simulink model "autosar_swc_expfcns"  (R2022b)
settings: Solver=FixedStepDiscrete  StartTime=0.0  StopTime=0.025  FixedStep=1  MaxStep=.0001  RelTol=1e-3  EnableMultiTasking=on
undefined symbols (not defined in the file): DiscIntNeverNeededParam
settings Model: Creator=The MathWorks, Inc.  LastModifiedBy=The MathWorks, Inc.
settings SolverCC: AlgebraicLoopSolver=TrustRegion  MaxZcPerStep=1
settings DataIOCC: LimitDataPoints=on  SaveFormat=Array  SaveOutput=off  SaveTime=off  ReturnWorkspaceOutputs=off
settings OptimizationCC: DefaultParameterBehavior=Inlined  InlineInvariantSignals=on  EnhancedBackFolding=on  ExpressionDepthLimit=2147483647  StateBitsets=on  DataBitsets=on  ZeroExternalMemoryAtStartup=off  ZeroInternalMemoryAtStartup=off  NoFixptDivByZeroProtection=on  EfficientFloat2IntCast=on  EfficientMapNaN2IntZero=off  LifeSpan=1  BufferReusableBoundary=off  EfficientTunableParamExpr=on
settings DebuggingCC: SigSpecEnsureSampleTimeMsg=none  UnconnectedInputMsg=warning  UnconnectedOutputMsg=warning  UnconnectedLineMsg=warning  BusObjectLabelMismatch=none  AllowSymbolicDim=off  StateNameClashWarn=warning  PregeneratedLibrarySubsystemCodeDiagnostic=none  StrictBusMsg=ErrorOnBusTreatedAsVector  SFUnexpectedBacktrackingDiag=warning  SFNoUnconditionalDefaultTransitionDiag=warning  SFExecutionAtInitializationDiag=none  SFMachineParentedDataDiag=warning  ArithmeticOperatorsInVariantConditions=warning
settings HardwareCC: ProdLongLongMode=on  TargetIntDivRoundTo=Zero  TargetEndianess=LittleEndian  TargetHWDeviceType=Generic->32-bit Embedded Processor
settings ModelReferenceCC: EnableRefExpFcnMdlSchedulingChecks=on  ModelReferenceNumInstancesAllowed=Single  PropagateSignalLabelsOutOfModel=off
settings SFSimCC: SimUseLocalCustomCode=off  SimParseCustomCode=off  CustomCodeUndefinedFunction=UseInterfaceOnly
settings RTWCC: Description=AUTOSAR  SystemTargetFile=autosar.tlc  GenCodeOnly=on  TemplateMakefile=ert_default_tmf  GenerateReport=on  RTWVerbose=off  RTWUseLocalCustomCode=off  IncludeHyperlinkInReport=on  LaunchReport=on  PortableWordSizes=on  DLArmComputeVersion=19.05
settings CodeAppCC: ForceParamTrailComments=on  IgnoreCustomStorageClasses=off  IgnoreTestpoints=on  SimulinkDataObjDesc=on  CustomSymbolStrGlobalVar=rt$N$M  CustomSymbolStrType=$N$M  CustomSymbolStrFcn=$N$M$F  CustomSymbolStrMacro=$N$M  InsertBlockDesc=on  StateflowObjectComments=on  InternalIdentifier=Classic
settings STFCustomTargetCC: UtilityFuncGeneration=Shared location  ParMdlRefBuildCompliant=on  CompOptLevelCompliant=on  IncludeMdlTerminateFcn=off  CombineOutputUpdateFcns=on  SuppressErrorStatus=on  ERTCustomFileBanners=on  SupportNonFinite=off  SupportComplex=off  SupportContinuousTime=off  SupportNonInlinedSFcns=off  RemoveResetFunc=on  MATLABClassNameForMDSCustomization=Simulink.SoftwareTarget.ERTCustomization  CPPClassGenCompliant=on  AutosarCompliant=on  UseToolchainInfoCompliant=on  LookupTableObjectStructAxisOrder=2,1,3,4,...  LUTObjectStructOrderEvenSpacing=Size,Table,Breakpoints  SystemTargetFile=autosar.tlc
settings ERTTargetCC: UtilityFuncGeneration=Shared location  MultiwordLength=2048  ConcurrentExecutionCompliant=off  IncludeMdlTerminateFcn=off  SuppressErrorStatus=on  SupportNonFinite=off  SupportComplex=off  ModelStepFunctionPrototypeControlCompliant=off  AutosarCompliant=on  LookupTableObjectStructAxisOrder=2,1,3,4,...  LUTObjectStructOrderEvenSpacing=Size,Table,Breakpoints  ExtModeMexFile=noextcomm  InlinedParameterPlacement=NonHierarchical  ERTCustomFileTemplate=example_file_process.tlc  ERTFilePackagingFormat=CompactWithDataFile  ConvertIfToSwitch=off  SuppressUnreachableDefaultCases=off
settings ConfigComp: CovMetricSettings=dw  CovSaveCumulativeToWorkspaceVar=on  CovSaveSingleToWorkspaceVar=on  CovExternalEMLEnable=off

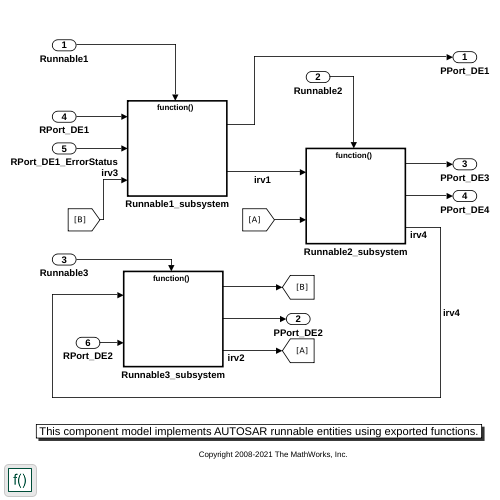
[thumbnail: Simulink's stored preview of the top-level diagram]
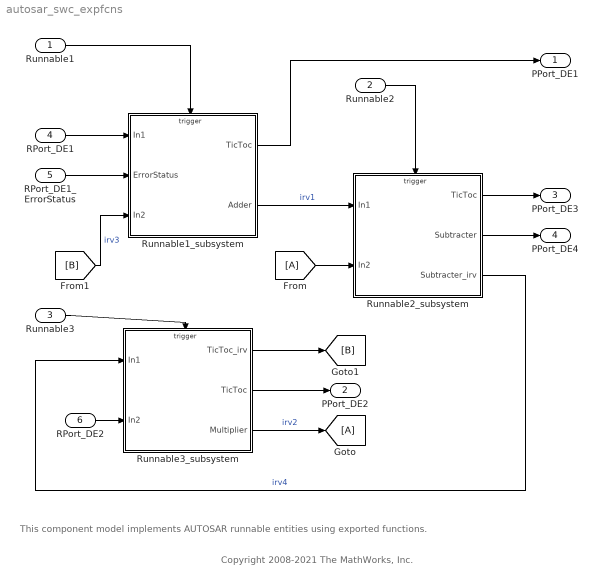
== system autosar_swc_expfcns ==
  note: This component model implements AUTOSAR runnable entities using exported functions.
  note: Copyright 2008-2021 The MathWorks, Inc.
  Runnable1 : Inport  PortDimensions=1  SampleTime=1  OutputFunctionCall=on
  Runnable2 : Inport  Port=2  PortDimensions=1  SampleTime=1  OutputFunctionCall=on
  Runnable3 : Inport  Port=3  PortDimensions=1  SampleTime=10  OutputFunctionCall=on
  RPort_DE1 : Inport  Port=4  OutDataTypeStr=double  PortDimensions=1
  RPort_DE1_ErrorStatus : Inport  Port=5  OutDataTypeStr=uint8  PortDimensions=1
  RPort_DE2 : Inport  Port=6  OutDataTypeStr=double  PortDimensions=2
  From : From
  Goto : Goto
  Runnable1_subsystem : Subsystem  TreatAsAtomicUnit=on  RTWFcnName=foo
  Runnable2_subsystem : Subsystem  TreatAsAtomicUnit=on  RTWFcnName=foo
  Runnable3_subsystem : Subsystem  TreatAsAtomicUnit=on  RTWFcnName=foo
  PPort_DE1 : Outport  OutDataTypeStr=int8  PortDimensions=1  VectorParamsAs1DForOutWhenUnconnected=off
  PPort_DE2 : Outport  Port=2  OutDataTypeStr=int8  PortDimensions=1  VectorParamsAs1DForOutWhenUnconnected=off
  PPort_DE3 : Outport  Port=3  OutDataTypeStr=int8  PortDimensions=2  VectorParamsAs1DForOutWhenUnconnected=off
  PPort_DE4 : Outport  Port=4  OutDataTypeStr=double  PortDimensions=1  VectorParamsAs1DForOutWhenUnconnected=off
  wires:
  [B] -> Runnable1_subsystem/3(In2)  "irv3"
  Runnable3_subsystem/1(TicToc_irv) -> [B]
  From/1 -> Runnable2_subsystem/2(In2)
  Runnable3_subsystem/3(Multiplier) -> Goto/1  "irv2"
  RPort_DE1_ErrorStatus/1 -> Runnable1_subsystem/2(ErrorStatus)
  Runnable2_subsystem/2(Subtracter) -> PPort_DE4/1
  RPort_DE1/1 -> Runnable1_subsystem/1(In1)
  Runnable2/1 -> Runnable2_subsystem/Trigger
  Runnable1_subsystem/1(TicToc) -> PPort_DE1/1
  Runnable2_subsystem/1(TicToc) -> PPort_DE3/1
  Runnable3_subsystem/2(TicToc) -> PPort_DE2/1
  Runnable1/1 -> Runnable1_subsystem/Trigger
  Runnable1_subsystem/2(Adder) -> Runnable2_subsystem/1(In1)  "irv1"
  Runnable2_subsystem/3(Subtracter_irv) -> Runnable3_subsystem/1(In1)  "irv4"
  RPort_DE2/1 -> Runnable3_subsystem/2(In2)
  Runnable3/1 -> Runnable3_subsystem/Trigger

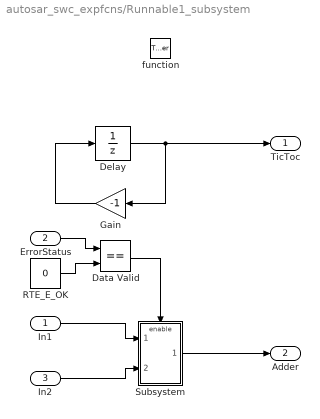
== system autosar_swc_expfcns/Runnable1_subsystem ==
  In1 : Inport
  ErrorStatus : Inport  Port=2
  In2 : Inport  Port=3
  function : TriggerPort  TriggerType=function-call  VariantControl=Variant  SampleTimeType=periodic  SampleTime=-1
  Data Valid : RelationalOperator  Operator===  OutDataTypeStr=boolean  InputSameDT=off
  Delay : UnitDelay  InitialCondition=1  SampleTime=-1  HasFrameUpgradeWarning=on
  Gain : Gain  Gain=-1  OutDataTypeStr=fixdt(1,8,0)
  RTE_E_OK : Constant  Value=0
  Subsystem : Subsystem
  TicToc : Outport  InitialOutput=0  VectorParamsAs1DForOutWhenUnconnected=off
  Adder : Outport  Port=2  InitialOutput=0  VectorParamsAs1DForOutWhenUnconnected=off
  wires:
  RTE_E_OK/1 -> Data Valid/2
  ErrorStatus/1 -> Data Valid/1
  Data Valid/1 -> Subsystem/Enable
  In2/1 -> Subsystem/2(In2)
  In1/1 -> Subsystem/1(In1)
  Delay/1 -> Gain/1, TicToc/1
  Gain/1 -> Delay/1
  Subsystem/1(Out1) -> Adder/1

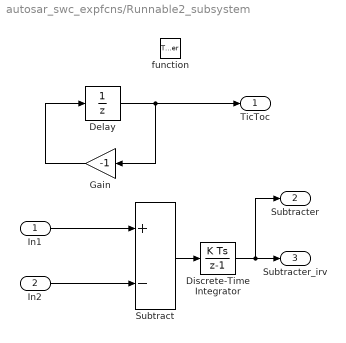
== system autosar_swc_expfcns/Runnable2_subsystem ==
  In1 : Inport
  In2 : Inport  Port=2
  function : TriggerPort  TriggerType=function-call  VariantControl=Variant  SampleTimeType=periodic  SampleTime=-1
  Delay : UnitDelay  InitialCondition=1  SampleTime=-1  HasFrameUpgradeWarning=on
  Discrete-Time Integrator : DiscreteIntegrator  SampleTime=-1  ICPrevOutput=DiscIntNeverNeededParam  ICPrevScaledInput=DiscIntNeverNeededParam
  Gain : Gain  Gain=-1  OutDataTypeStr=fixdt(1,8,0)
  Subtract : Sum  Inputs=+-
  TicToc : Outport  InitialOutput=0  VectorParamsAs1DForOutWhenUnconnected=off
  Subtracter : Outport  Port=2  InitialOutput=0  VectorParamsAs1DForOutWhenUnconnected=off
  Subtracter_irv : Outport  Port=3  VectorParamsAs1DForOutWhenUnconnected=off
  wires:
  Discrete-Time Integrator/1 -> Subtracter/1, Subtracter_irv/1
  Subtract/1 -> Discrete-Time Integrator/1
  Gain/1 -> Delay/1
  Delay/1 -> TicToc/1, Gain/1
  In1/1 -> Subtract/1
  In2/1 -> Subtract/2

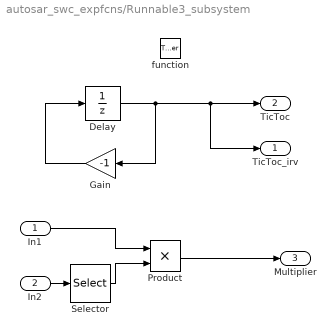
== system autosar_swc_expfcns/Runnable3_subsystem ==
  In1 : Inport  OutDataTypeStr=double
  In2 : Inport  Port=2
  function : TriggerPort  TriggerType=function-call  VariantControl=Variant  SampleTimeType=periodic  SampleTime=-1
  Delay : UnitDelay  InitialCondition=1  SampleTime=-1  HasFrameUpgradeWarning=on
  Gain : Gain  Gain=-1  OutDataTypeStr=fixdt(1,8,0)
  Product : Product  Inputs=**  OutDataTypeStr=Inherit: Same as first input
  Selector : Selector  InputPortWidth=2  IndexOptions=Index vector (dialog)  Indices=1  OutputSizes=1
  TicToc_irv : Outport  VectorParamsAs1DForOutWhenUnconnected=off
  TicToc : Outport  Port=2  InitialOutput=0  VectorParamsAs1DForOutWhenUnconnected=off
  Multiplier : Outport  Port=3  InitialOutput=0  VectorParamsAs1DForOutWhenUnconnected=off
  wires:
  Selector/1 -> Product/2
  Product/1 -> Multiplier/1
  Gain/1 -> Delay/1
  Delay/1 -> TicToc_irv/1, TicToc/1, Gain/1
  In1/1 -> Product/1
  In2/1 -> Selector/1

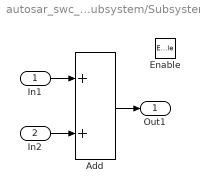
== system autosar_swc_expfcns/Runnable1_subsystem/Subsystem ==
  In1 : Inport
  In2 : Inport  Port=2
  Enable : EnablePort
  Add : Sum
  Out1 : Outport  VectorParamsAs1DForOutWhenUnconnected=off
  wires:
  In2/1 -> Add/2
  Add/1 -> Out1/1
  In1/1 -> Add/1
